simulink model "L1_2"  (R2017b)
settings: Solver=ode4  StartTime=0.0  StopTime=30  FixedStep=0.01  RelTol=1e-3
libraries: simulink x7
settings Model: Creator=tutuc  LastModifiedBy=tutuc

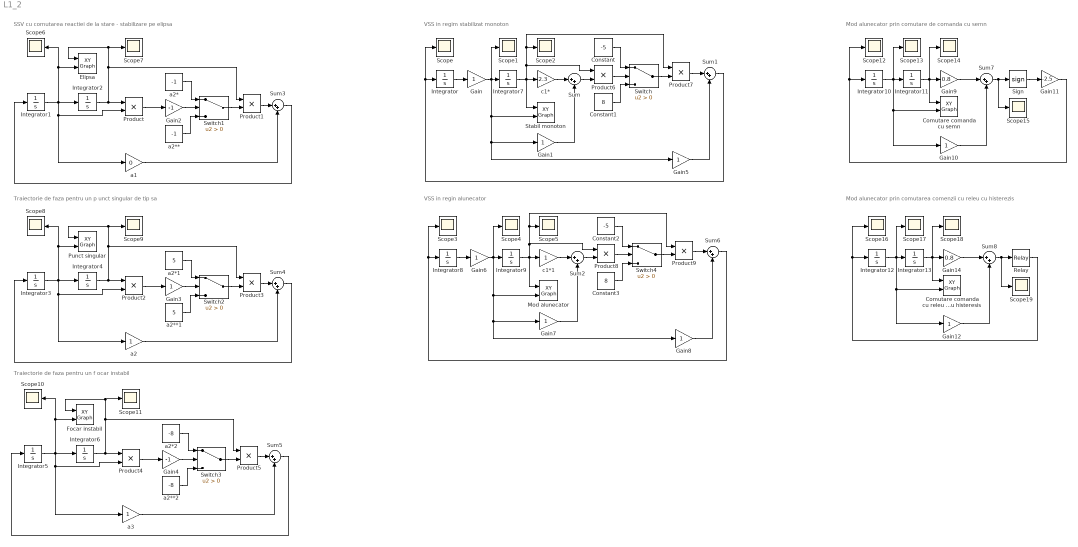
== system L1_2 ==
  note: Mod alunecator prin comutarea comenzii cu releu cu histerezis
  note: Mod alunecator prin comutare de comanda cu semn
  note: VSS in regin alunecator
  note: VSS in regim stabilizat monoton
  note: Traiectorie de faza pentru un f ocar instabil
  note: Traiectorie de faza pentru un p unct singular de tip sa
  note: SSV cu comutarea reactiei de la stare - stabilizare pe elipsa
  Comutare comanda cu releu cu histeresis : simulink/Sinks/XY Graph  xmin=-100  xmax=100  ymin=-10  ymax=20  st=-1
  Comutare comanda cu semn : simulink/Sinks/XY Graph  xmin=-15  xmax=3  ymin=-10  ymax=10  st=-1
  Constant : Constant  Value=-5
  Constant1 : Constant  Value=8
  Constant2 : Constant  Value=-5
  Constant3 : Constant  Value=8
  Elipsa : simulink/Sinks/XY Graph  xmin=-10  xmax=10  ymin=-10  ymax=10  st=-1
  Focar instabil : simulink/Sinks/XY Graph  xmin=-150  xmax=150  ymin=-300  ymax=300  st=-1
  Gain{,1,3,5..8,10,12} (9 alike) : Gain
  Gain11 : Gain  Gain=-2.5
  Gain14 : Gain  Gain=0.8
  Gain2 : Gain  Gain=-1
  Gain4 : Gain  Gain=-1
  Gain9 : Gain  Gain=0.8
  Integrator{,7..11} (6 alike) : Integrator  InitialCondition=-5
  Integrator{1..6,12} (7 alike) : Integrator  InitialCondition=3
  Integrator13 : Integrator  InitialCondition=2
  Mod alunecator : simulink/Sinks/XY Graph  xmin=-10  xmax=10  ymin=-10  ymax=10  st=-1
  Product{,1..9} (10 alike) : Product
  Punct singular : simulink/Sinks/XY Graph  xmin=-5  xmax=100  ymin=-5  ymax=250  st=-1
  Relay : Relay  OnSwitchValue=0.1  OffSwitchValue=0.1
  Scope{,1..19} (20 alike) : Scope
  Sign : Signum
  Stabil monoton : simulink/Sinks/XY Graph  xmin=-10  xmax=10  ymin=-10  ymax=10  st=-1
  Sum{,1..8} (9 alike) : Sum  Inputs=|++
  Switch{,1..4} (5 alike) : Switch  Criteria=u2 > Threshold
  a1 : Gain  Gain=0
  a2 : Gain
  a2* : Constant  Value=-1
  a2** : Constant  Value=-1
  a2**1 : Constant  Value=5
  a2**2 : Constant  Value=-8
  a2*1 : Constant  Value=5
  a2*2 : Constant  Value=-8
  a3 : Gain
  c1* : Gain  Gain=2.3
  c1*1 : Gain
  wires:
  Integrator1/1 -> Elipsa/2, Scope6/1, a1/1, Product/2, Integrator2/1
  Integrator2/1 -> Elipsa/1, Scope7/1, Product1/1, Product/1
  Product/1 -> Gain2/1
  Gain2/1 -> Switch1/2
  a2*/1 -> Switch1/1
  a2**/1 -> Switch1/3
  Switch1/1 -> Product1/2
  Product1/1 -> Sum3/1
  Sum3/1 -> Integrator1/1
  a1/1 -> Sum3/2
  a2/1 -> Sum4/2
  Sum4/1 -> Integrator3/1
  Product3/1 -> Sum4/1
  Switch2/1 -> Product3/2
  a2**1/1 -> Switch2/3
  a2*1/1 -> Switch2/1
  Gain3/1 -> Switch2/2
  Product2/1 -> Gain3/1
  Integrator4/1 -> Product2/1, Product3/1, Scope9/1, Punct singular/1
  Integrator3/1 -> Integrator4/1, Product2/2, a2/1, Scope8/1, Punct singular/2
  Integrator5/1 -> Focar instabil/2, Scope10/1, a3/1, Product4/2, Integrator6/1
  Integrator6/1 -> Focar instabil/1, Scope11/1, Product5/1, Product4/1
  Product4/1 -> Gain4/1
  Gain4/1 -> Switch3/2
  a2*2/1 -> Switch3/1
  a2**2/1 -> Switch3/3
  Switch3/1 -> Product5/2
  Product5/1 -> Sum5/1
  Sum5/1 -> Integrator5/1
  a3/1 -> Sum5/2
  Integrator/1 -> Gain/1
  Gain/1 -> Stabil monoton/2, Gain5/1, Gain1/1, Scope1/1, Integrator7/1
  Integrator7/1 -> Product6/1, Product7/1, Scope2/1, Stabil monoton/1, c1*/1
  c1*/1 -> Sum/1
  Gain1/1 -> Sum/2
  Sum/1 -> Product6/2
  Product6/1 -> Switch/2
  Constant/1 -> Switch/1
  Constant1/1 -> Switch/3
  Switch/1 -> Product7/2
  Product7/1 -> Sum1/1
  Gain5/1 -> Sum1/2
  Sum1/1 -> Scope/1, Integrator/1
  Sum6/1 -> Integrator8/1, Scope3/1
  Gain8/1 -> Sum6/2
  Product9/1 -> Sum6/1
  Switch4/1 -> Product9/2
  Constant3/1 -> Switch4/3
  Constant2/1 -> Switch4/1
  Product8/1 -> Switch4/2
  Sum2/1 -> Product8/2
  Gain7/1 -> Sum2/2
  c1*1/1 -> Sum2/1
  Integrator9/1 -> c1*1/1, Mod alunecator/1, Scope5/1, Product9/1, Product8/1
  Gain6/1 -> Integrator9/1, Scope4/1, Gain7/1, Gain8/1, Mod alunecator/2
  Integrator8/1 -> Gain6/1
  Integrator10/1 -> Gain10/1, Comutare comanda cu semn/2, Scope13/1, Integrator11/1
  Integrator11/1 -> Scope14/1, Comutare comanda cu semn/1, Gain9/1
  Gain9/1 -> Sum7/1
  Gain10/1 -> Sum7/2
  Sum7/1 -> Scope15/1, Sign/1
  Sign/1 -> Gain11/1
  Gain11/1 -> Scope12/1, Integrator10/1
  Relay/1 -> Integrator12/1, Scope16/1
  Sum8/1 -> Relay/1, Scope19/1
  Gain12/1 -> Sum8/2
  Gain14/1 -> Sum8/1
  Integrator13/1 -> Gain14/1, Comutare comanda cu releu cu histeresis/1, Scope18/1
  Integrator12/1 -> Integrator13/1, Scope17/1, Comutare comanda cu releu cu histeresis/2, Gain12/1
